simulink model "gps_estimate_dop_demo"  (Simulink 7.3)
settings: Solver=ode45  StartTime=0.0  StopTime=86400  RelTol=1e-3
undefined symbols (not defined in the file): WGS
libraries: rapidstm32_gps_lib x3
settings Model: Creator=Compaq  LastModifiedBy=Compaq

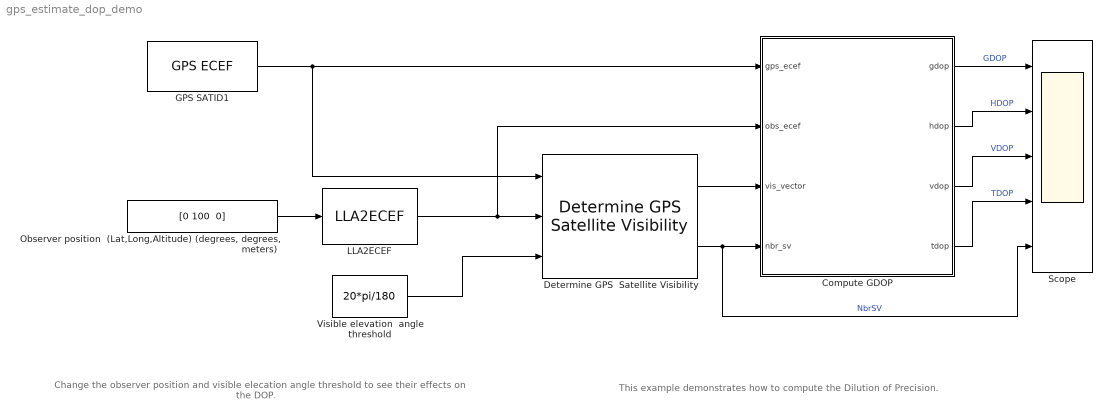
== system gps_estimate_dop_demo ==
  note: This example demonstrates how to compute the Dilution of Precision.
  note: Change the observer position
      | and visible elecation angle threshold
      | to see their effects on the DOP.
  Compute GDOP : Stateflow chart
  Determine GPS  Satellite Visibility : rapidstm32_gps_lib/Determine GPS  Satellite Visibility
  GPS SATID1 : rapidstm32_gps_lib/GPS ECEF  satid=All 24  t0=0  sampletime=30
  LLA2ECEF : rapidstm32_gps_lib/LLA2ECEF  latlong_format=Degrees  refellipsoid=WGS-84  re=6378137  epsilon=0.081819190842622
  "Observer position  (Lat,Long,Altitude) (degrees, degrees, meters)" : Constant  Value="[0 100  0]"  OutDataType=fixdt(1, 16)  OutScaling=2^0
  Scope : Scope  NumInputPorts=5
      settings: TimeRange=86400  YMin=1~0~0~-8.67362e-019~1  YMax=8~30~25~0.03~4
  Visible elevation  angle threshold : Constant  Value=20*pi/180  OutDataType=fixdt(1, 16)  OutScaling=2^0
  wires:
  GPS SATID1/1 -> Determine GPS  Satellite Visibility/1, Compute GDOP/1(gps_ecef)
  "Observer position  (Lat,Long,Altitude) (degrees, degrees, meters)"/1 -> LLA2ECEF/1
  LLA2ECEF/1 -> Determine GPS  Satellite Visibility/2, Compute GDOP/2(obs_ecef)
  Visible elevation  angle threshold/1 -> Determine GPS  Satellite Visibility/3
  Determine GPS  Satellite Visibility/2 -> Compute GDOP/4(nbr_sv), Scope/5  "NbrSV"
  Determine GPS  Satellite Visibility/1 -> Compute GDOP/3(vis_vector)
  Compute GDOP/1(gdop) -> Scope/1  "GDOP"
  Compute GDOP/2(hdop) -> Scope/2  "HDOP"
  Compute GDOP/3(vdop) -> Scope/3  "VDOP"
  Compute GDOP/4(tdop) -> Scope/4  "TDOP"

== matlab function Compute GDOP ==
  data: gps_ecef input double; obs_ecef input double; vis_vector input double; gdop output double; nbr_sv input double; hdop output double; vdop output double; tdop output double
function [gdop, hdop, vdop, tdop] = compute_dop(gps_ecef, obs_ecef, vis_vector, nbr_sv)
%#eml

% This algorithm is not yet optimized due to limitation of the Embedded
% MATLAB function block which does not allow for dynamic vector/matrix indexing.
% So G is still a 24-by-4 matrix even if not all satellites are visible.

G = [zeros(24,3) ones(24,1)];
idx = 1;
for i = 1:24
    if (vis_vector(i) == 1)
        unit_vector = gps_ecef(:,i) - obs_ecef;
        r = sqrt(sum(unit_vector.^2,1));
        G(idx,1:3) = -unit_vector'./r;
        idx = idx + 1;
    end
end
if (idx >= 4)
    dop = inv(G'*G); % to be optimized
    gdop = sqrt(trace(dop));
    hdop = sqrt(sum(dop(1:2).^2));
    vdop = sqrt(dop(3).^2);
    tdop = sqrt(dop(4).^2);
else
    gdop = NaN;
    hdop = NaN;
    vdop = NaN;
    tdop = NaN;
end
